simulink model "PRACTICALA"  (R2023a)
settings: Solver=ode15s  StartTime=0.0  StopTime=5  MaxStep=1e-3  RelTol=1e-3
settings Model: Creator=piqui  LastModifiedBy=jaelb
settings DataIOCC: ReturnWorkspaceOutputs=off  TimeSaveName=t
settings DebuggingCC: AlgebraicLoopMsg=none  ArtificialAlgebraicLoopMsg=none  BlockPriorityViolationMsg=error  MinStepSizeMsg=error  MaxConsecutiveZCsMsg=none  ModelReferenceExtraNoncontSigs=none  OperatingPointInterfaceChecksumMismatchMsg=error

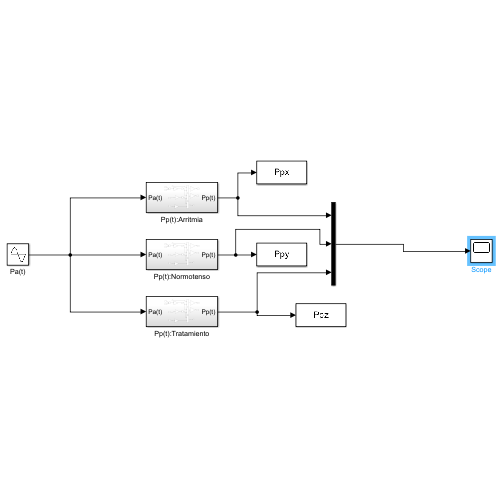
[thumbnail: Simulink's stored preview of the top-level diagram]
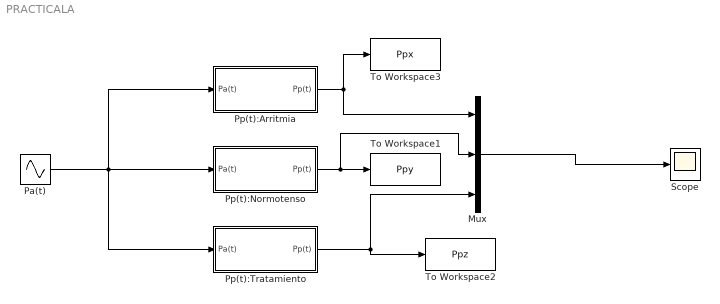
== system PRACTICALA ==
  Mux : Mux  Inputs=3
  Pa(t) : Sin  Frequency=2*pi  SampleTime=0
  Pp(t):Arritmia : Subsystem
  Pp(t):Normotenso : Subsystem
  Pp(t):Tratamiento : Subsystem
  Scope : Scope
  To Workspace1 : ToWorkspace  VariableName=Ppy  SampleTime=-1
  To Workspace2 : ToWorkspace  VariableName=Ppz  SampleTime=-1
  To Workspace3 : ToWorkspace  VariableName=Ppx  SampleTime=-1
  wires:
  Mux/1 -> Scope/1
  Pa(t)/1 -> Pp(t):Tratamiento/1(Pa(t)), Pp(t):Normotenso/1(Pa(t)), Pp(t):Arritmia/1(Pa(t))
  Pp(t):Arritmia/1(Pp(t)) -> Mux/1, To Workspace3/1
  Pp(t):Normotenso/1(Pp(t)) -> Mux/2, To Workspace1/1
  Pp(t):Tratamiento/1(Pp(t)) -> To Workspace2/1, Mux/3

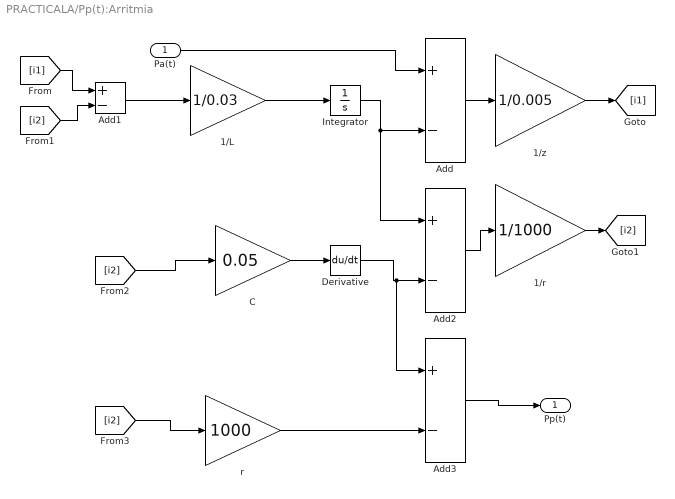
== system PRACTICALA/Pp(t):Arritmia ==
  Pa(t) : Inport
  1/L : Gain  Gain=1/0.03
  1/r : Gain  Gain=1/1000
  1/z : Gain  Gain=1/0.005
  Add{,1..3} (4 alike) : Sum  Inputs=+-
  C : Gain  Gain=0.05
  Derivative : Derivative
  Integrator : Integrator
  r : Gain  Gain=1000
  Pp(t) : Outport
  wires:
  [i2] -> r/1
  Pa(t)/1 -> Add/1
  r/1 -> Add3/2
  1/r/1 -> [i2]
  [i2] -> C/1
  1/L/1 -> Integrator/1
  Add3/1 -> Pp(t)/1
  Derivative/1 -> Add3/1, Add2/2
  C/1 -> Derivative/1
  Add/1 -> 1/z/1
  Add1/1 -> 1/L/1
  Add2/1 -> 1/r/1
  Integrator/1 -> Add2/1, Add/2
  1/z/1 -> [i1]
  [i2] -> Add1/2
  [i1] -> Add1/1

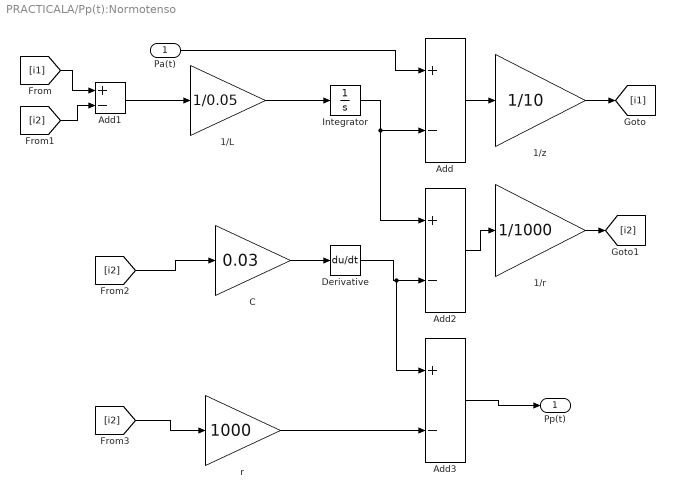
== system PRACTICALA/Pp(t):Normotenso ==
  Pa(t) : Inport
  1/L : Gain  Gain=1/0.05
  1/r : Gain  Gain=1/1000
  1/z : Gain  Gain=1/10
  Add{,1..3} (4 alike) : Sum  Inputs=+-
  C : Gain  Gain=0.03
  Derivative : Derivative
  Integrator : Integrator
  r : Gain  Gain=1000
  Pp(t) : Outport
  wires:
  Derivative/1 -> Add3/1, Add2/2
  C/1 -> Derivative/1
  1/z/1 -> [i1]
  r/1 -> Add3/2
  Add3/1 -> Pp(t)/1
  Add/1 -> 1/z/1
  Add2/1 -> 1/r/1
  Pa(t)/1 -> Add/1
  [i2] -> Add1/2
  Integrator/1 -> Add2/1, Add/2
  [i1] -> Add1/1
  [i2] -> r/1
  [i2] -> C/1
  1/L/1 -> Integrator/1
  1/r/1 -> [i2]
  Add1/1 -> 1/L/1

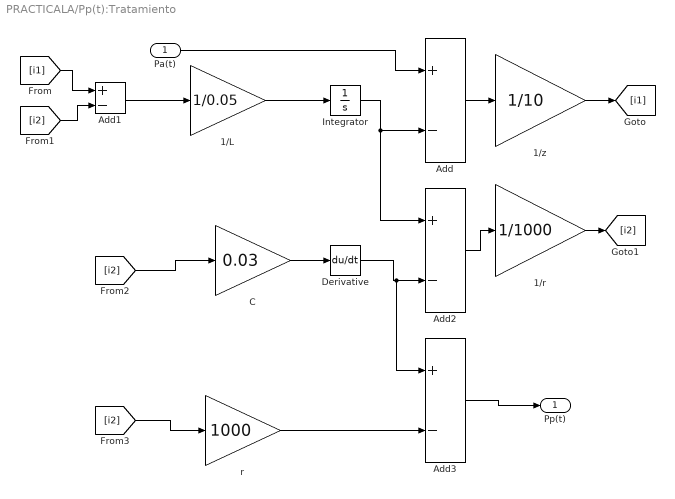
== system PRACTICALA/Pp(t):Tratamiento ==
  Pa(t) : Inport
  1/L : Gain  Gain=1/0.05
  1/r : Gain  Gain=1/1000
  1/z : Gain  Gain=1/10
  Add{,1..3} (4 alike) : Sum  Inputs=+-
  C : Gain  Gain=0.03
  Derivative : Derivative
  Integrator : Integrator
  r : Gain  Gain=1000
  Pp(t) : Outport
  wires:
  [i2] -> C/1
  Add/1 -> 1/z/1
  [i1] -> Add1/1
  Add2/1 -> 1/r/1
  1/L/1 -> Integrator/1
  1/z/1 -> [i1]
  Pa(t)/1 -> Add/1
  r/1 -> Add3/2
  [i2] -> Add1/2
  1/r/1 -> [i2]
  Integrator/1 -> Add2/1, Add/2
  [i2] -> r/1
  Add1/1 -> 1/L/1
  Add3/1 -> Pp(t)/1
  C/1 -> Derivative/1
  Derivative/1 -> Add3/1, Add2/2
